simulink model "test_angle_joint"  (Simulink 8.7)
settings: Solver=ode45  StartTime=0.0  StopTime=2  MaxStep=Step_Time  RelTol=1e-3
settings Model: Creator=saeed  LastModifiedBy=Other
settings DataIOCC: SignalLoggingSaveFormat=ModelDataLogs
settings OptimizationCC: ExpressionDepthLimit=2147483647
settings DebuggingCC: SolverPrmCheckMsg=warning  FcnCallInpInsideContextMsg=UseLocalSettings  StateNameClashWarn=warning
settings GRTTargetCC: CombineOutputUpdateFcns=off  GRTInterface=on
settings ConfigComp: CovSFcnEnable=off

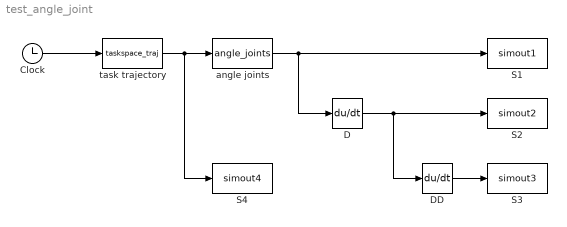
== system test_angle_joint ==
  Clock : Clock
  D : Derivative
  DD : Derivative
  S1 : ToWorkspace  VariableName=simout1  SaveFormat=Structure With Time  SampleTime=-1
  S2 : ToWorkspace  VariableName=simout2  SaveFormat=Structure With Time  SampleTime=-1
  S3 : ToWorkspace  VariableName=simout3  SaveFormat=Structure With Time  SampleTime=-1
  S4 : ToWorkspace  VariableName=simout4  SaveFormat=Structure With Time  SampleTime=-1
  angle joints : MATLABFcn  MATLABFcn=angle_joints
  task trajectory : MATLABFcn  MATLABFcn=taskspace_traj
  wires:
  Clock/1 -> task trajectory/1
  task trajectory/1 -> S4/1, angle joints/1
  angle joints/1 -> D/1, S1/1
  D/1 -> DD/1, S2/1
  DD/1 -> S3/1
